simulink model "disturbances"  (Simulink 6.3)
settings: Solver=ode45  StartTime=0.0  StopTime=10.0  RelTol=1e-3
libraries: aerolibutil x4, simulink x1
settings Model: LastModifiedBy=artur

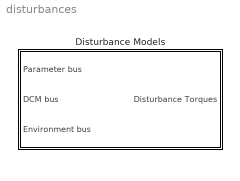
== system disturbances ==
  Disturbance Models : Subsystem

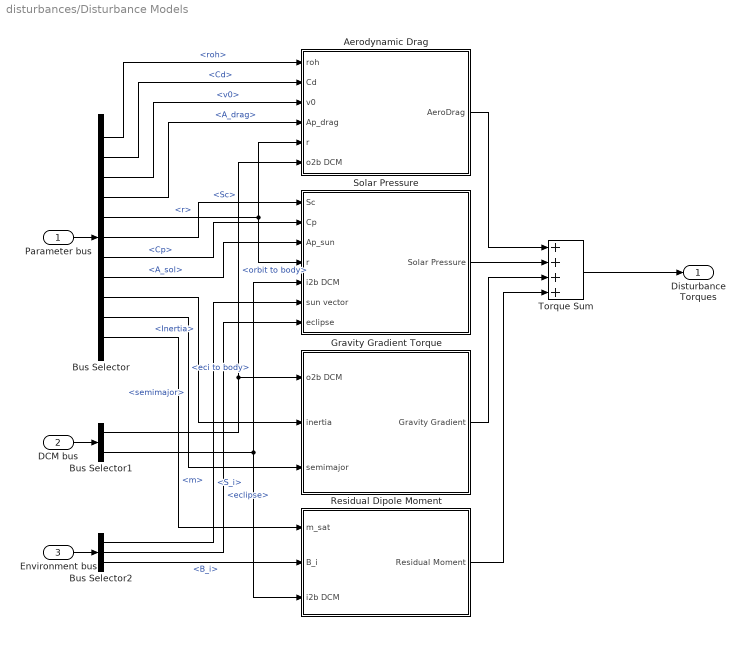
== system disturbances/Disturbance Models ==
  Parameter bus : Inport
  DCM bus : Inport  Port=2
  Environment bus : Inport  Port=3
  Aerodynamic Drag : Subsystem
  Bus Selector : BusSelector  OutputSignals=Orbit Parameters.roh,Satellite Parameters.Cd,Orbit Parameters.v0,Satellite Parameters.A_drag,Satellite Parameters.r,Orbit Parameters.Sc,Satellite Parameters.Cp,Satellite Parameters.A_sol,Satellite Parameters.Inertia,Orbit Parameters.semimajor,Satellite Parameters.m
  Bus Selector1 : BusSelector  OutputSignals=orbit to body,eci to body
  Bus Selector2 : BusSelector  OutputSignals=Sun Model.S_i,Sun Model.eclipse,Magnetic Field Model.B_i
  Gravity Gradient Torque : Subsystem
  Residual Dipole Moment : Subsystem
  Solar Pressure : Subsystem
  Torque Sum : Sum  Inputs=++++  OutScaling=2^-10
  Disturbance Torques : Outport
  wires:
  Aerodynamic Drag/1(AeroDrag) -> Torque Sum/1
  Parameter bus/1 -> Bus Selector/1
  Bus Selector/1 -> Aerodynamic Drag/1(roh)  "<roh>"
  Bus Selector/2 -> Aerodynamic Drag/2(Cd)  "<Cd>"
  Bus Selector/3 -> Aerodynamic Drag/3(v0)  "<v0>"
  Bus Selector/4 -> Aerodynamic Drag/4(Ap_drag)  "<A_drag>"
  Bus Selector/5 -> Aerodynamic Drag/5(r), Solar Pressure/4(r)  "<r>"
  Bus Selector/6 -> Solar Pressure/1(Sc)  "<Sc>"
  Bus Selector/7 -> Solar Pressure/2(Cp)  "<Cp>"
  Bus Selector/8 -> Solar Pressure/3(Ap_sun)  "<A_sol>"
  Bus Selector/9 -> Gravity Gradient Torque/2(inertia)  "<Inertia>"
  Bus Selector/10 -> Gravity Gradient Torque/3(semimajor)  "<semimajor>"
  Bus Selector/11 -> Residual Dipole Moment/1(m_sat)  "<m>"
  DCM bus/1 -> Bus Selector1/1
  Bus Selector1/1 -> Aerodynamic Drag/6(o2b DCM), Gravity Gradient Torque/1(o2b DCM)  "<orbit to body>"
  Bus Selector1/2 -> Solar Pressure/5(i2b DCM), Residual Dipole Moment/3(i2b DCM)  "<eci to body>"
  Gravity Gradient Torque/1(Gravity Gradient) -> Torque Sum/3
  Environment bus/1 -> Bus Selector2/1
  Bus Selector2/1 -> Solar Pressure/6(sun vector)  "<S_i>"
  Bus Selector2/2 -> Solar Pressure/7(eclipse)  "<eclipse>"
  Bus Selector2/3 -> Residual Dipole Moment/2(B_i)  "<B_i>"
  Solar Pressure/1(Solar Pressure) -> Torque Sum/2
  Torque Sum/1 -> Disturbance Torques/1
  Residual Dipole Moment/1(Residual Moment) -> Torque Sum/4

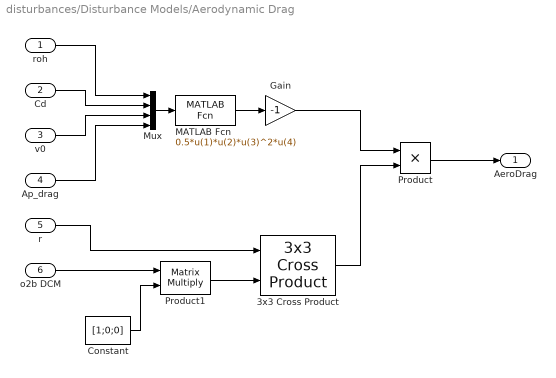
== system disturbances/Disturbance Models/Aerodynamic Drag ==
  roh : Inport
  Cd : Inport  Port=2
  v0 : Inport  Port=3
  Ap_drag : Inport  Port=4
  r : Inport  Port=5
  o2b DCM : Inport  Port=6
  3x3 Cross Product : aerolibutil/3x3 Cross Product
  Constant : Constant  Value=[1;0;0]
  Gain : Gain  Gain=-1
  MATLAB Fcn : MATLABFcn  MATLABFcn=0.5*u(1)*u(2)*u(3)^2*u(4)
  Mux : Mux
  Product : Product  RndMeth=Zero
  Product1 : Product  Multiplication=Matrix(*)  RndMeth=Zero
  AeroDrag : Outport
  wires:
  Mux/1 -> MATLAB Fcn/1
  roh/1 -> Mux/1
  Cd/1 -> Mux/2
  v0/1 -> Mux/3
  Ap_drag/1 -> Mux/4
  Constant/1 -> Product1/2
  o2b DCM/1 -> Product1/1
  Product1/1 -> 3x3 Cross Product/2
  r/1 -> 3x3 Cross Product/1
  MATLAB Fcn/1 -> Gain/1
  Gain/1 -> Product/1
  3x3 Cross Product/1 -> Product/2
  Product/1 -> AeroDrag/1

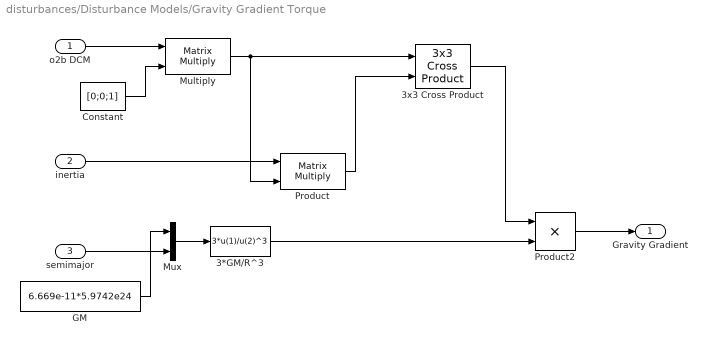
== system disturbances/Disturbance Models/Gravity Gradient Torque ==
  o2b DCM : Inport
  inertia : Inport  Port=2
  semimajor : Inport  Port=3
  3*GM/R^3 : MATLABFcn  MATLABFcn=3*u(1)/u(2)^3
  3x3 Cross Product : aerolibutil/3x3 Cross Product
  Constant : Constant  Value=[0;0;1]
  GM : Constant  Value=6.669e-11*5.9742e24
  Multiply : Product  Multiplication=Matrix(*)  RndMeth=Zero
  Mux : Mux  Inputs=2
  Product : Product  Multiplication=Matrix(*)  RndMeth=Zero
  Product2 : Product  RndMeth=Zero
  Gravity Gradient : Outport
  wires:
  Product/1 -> 3x3 Cross Product/2
  3x3 Cross Product/1 -> Product2/1
  Product2/1 -> Gravity Gradient/1
  o2b DCM/1 -> Multiply/1
  Constant/1 -> Multiply/2
  3*GM/R^3/1 -> Product2/2
  inertia/1 -> Product/1
  Multiply/1 -> Product/2, 3x3 Cross Product/1
  Mux/1 -> 3*GM/R^3/1
  semimajor/1 -> Mux/2
  GM/1 -> Mux/1

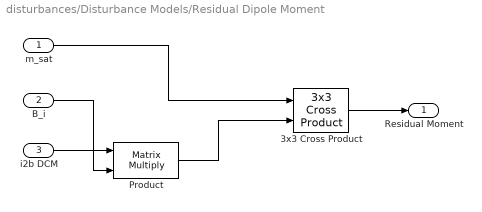
== system disturbances/Disturbance Models/Residual Dipole Moment ==
  m_sat : Inport
  B_i : Inport  Port=2
  i2b DCM : Inport  Port=3
  3x3 Cross Product : aerolibutil/3x3 Cross Product
  Product : Product  Multiplication=Matrix(*)  RndMeth=Zero
  Residual Moment : Outport
  wires:
  3x3 Cross Product/1 -> Residual Moment/1
  i2b DCM/1 -> Product/1
  B_i/1 -> Product/2
  m_sat/1 -> 3x3 Cross Product/1
  Product/1 -> 3x3 Cross Product/2

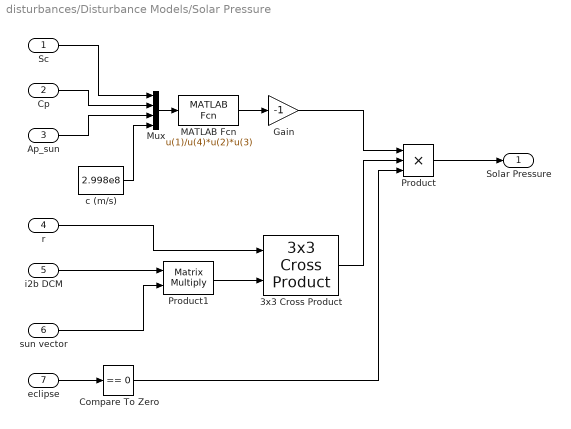
== system disturbances/Disturbance Models/Solar Pressure ==
  Sc : Inport
  Cp : Inport  Port=2
  Ap_sun : Inport  Port=3
  r : Inport  Port=4
  i2b DCM : Inport  Port=5
  sun vector : Inport  Port=6
  eclipse : Inport  Port=7
  3x3 Cross Product : aerolibutil/3x3 Cross Product
  Compare To Zero : simulink/Logic and Bit Operations/Compare To Zero  relop===  LogicOutDataTypeMode=uint8  ZeroCross=off
  Gain : Gain  Gain=-1
  MATLAB Fcn : MATLABFcn  MATLABFcn=u(1)/u(4)*u(2)*u(3)
  Mux : Mux
  Product : Product  Inputs=3  RndMeth=Zero
  Product1 : Product  Multiplication=Matrix(*)  RndMeth=Zero
  c (m/s) : Constant  Value=2.998e8
  Solar Pressure : Outport
  wires:
  Mux/1 -> MATLAB Fcn/1
  Sc/1 -> Mux/1
  Cp/1 -> Mux/2
  Ap_sun/1 -> Mux/3
  sun vector/1 -> Product1/2
  i2b DCM/1 -> Product1/1
  Product1/1 -> 3x3 Cross Product/2
  r/1 -> 3x3 Cross Product/1
  MATLAB Fcn/1 -> Gain/1
  Gain/1 -> Product/1
  3x3 Cross Product/1 -> Product/2
  Product/1 -> Solar Pressure/1
  c (m/s)/1 -> Mux/4
  eclipse/1 -> Compare To Zero/1
  Compare To Zero/1 -> Product/3
